simulink model "plantTest"  (R2024b)
settings: Solver=FixedStepAuto  StartTime=0.0  StopTime=50.0  FixedStep=.01  RelTol=1e-3
libraries: mpclib x1
settings Model: Creator=andre  LastModifiedBy=andre

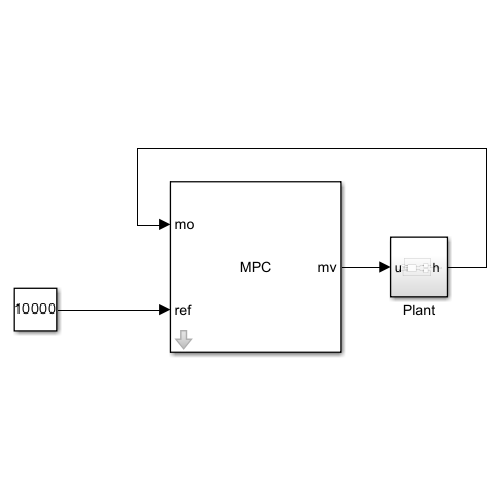
[thumbnail: Simulink's stored preview of the top-level diagram]
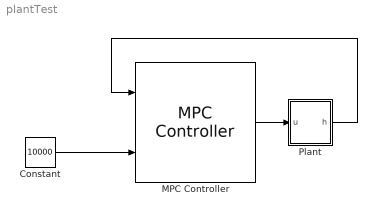
== system plantTest ==
  Constant : Constant  Value=10000
  MPC Controller : mpclib/MPC Controller  SCDEnableBlockLinearizationSpecification=on  is_multiple=0  enable_value=0  return_u0=off  updateMPCinCallerWorkspace=on  md_inport=off  mv_inport=off  uref_inport=off  return_cost=off  return_mvseq=off  return_qpstatus=off  return_xseq=off  return_state=off  return_ovseq=off  state_inport=off  umin_inport=off  umax_inport=off  ymin_inport=off  ymax_inport=off  cc_inport=off  ywt_inport=off  uwt_inport=off  duwt_inport=off  rhoeps_inport=off  pm_inport=off  MaximumP=80  HorizonChoice=FixedHorizon  n_ts=0.01  n_p=300  n_mv=1  n_md=1  n_ud=0  n_mo=1  n_uo=0  BlockDataType=double  SampleTimeInherited=off  switch_inport=off
  Plant : Subsystem
  wires:
  MPC Controller/1 -> Plant/1(u)
  Plant/1("h ") -> MPC Controller/1
  Constant/1 -> MPC Controller/2

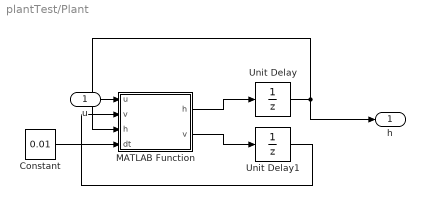
== system plantTest/Plant ==
  u : Inport
  Constant : Constant  Value=0.01
  MATLAB Function : MATLAB Function  TreatAsAtomicUnit=on
  Unit Delay : UnitDelay  InitialCondition=3851  SampleTime=-1  HasFrameUpgradeWarning=on
  Unit Delay1 : UnitDelay  InitialCondition=255.27  SampleTime=-1  HasFrameUpgradeWarning=on
  "h " : Outport
  wires:
  Constant/1 -> MATLAB Function/4(dt)
  Unit Delay/1 -> "h "/1, MATLAB Function/3("h ")
  Unit Delay1/1 -> MATLAB Function/2("v ")
  MATLAB Function/2(v) -> Unit Delay1/1
  MATLAB Function/1(h) -> Unit Delay/1
  u/1 -> MATLAB Function/1(u)

== matlab function plantTest/Plant/MATLAB Function ==
  data: u input; h output; v input; h input; dt input; v output
function [h,v] = fcn(u, v, h, dt)
    if (h <= 0)
        h = 0;
        v = 0;
        return;
    end

    m = 21.962;        % Mass of the rocket (kg)
    g = 9.81;          % Gravity (m/s^2)
    rho = 1.125;       % Air density (kg/m^3)
    A_brake = 0.0078;  % Cross-sectional area of airbrakes(m^2)
    Cd_brake = 1.1;    % Drag coefficient of airbrakes
    A_rocket = 0.0453; % Cross-sectional area (m^2)
    Cd_rocket = 0.413; % Drag coefficient of rocket
    v = v - ((9.81 + ((rho * v^(2) / (2 * m)) * (A_brake * Cd_brake * u + A_rocket * Cd_rocket / 3.14)))) * dt; % The division by pi is to lower the effect of drag, because it seems to high right now and I dont have time to firgure out why
    h = h + v * dt * 3.28084;
    disp("fdsafsafafda");
    disp(h);

    disp("1")
    disp((rho .* v^(2) ./ (2 .* m)));
    disp("2")
    disp(A_brake .* Cd_brake .* u);
    disp("3")    
    disp(A_rocket * Cd_rocket);
